simulink model "real_UIO_alternative_2021_02_17_02"  (R2019b)
settings: Solver=FixedStepAuto  StartTime=0.0  StopTime=60  FixedStep=0.01  RelTol=1e-3
values from neighbouring files (symbols this model uses):
  A = A-0.1*eye(2)    [DAC_UIO_Comp.m]    (also in LinearND_QUANTUM_2020_11_14_2.m = A+(basis{i}*rand()); UIO_adaptive_example.m = [-2379.2 0 0 0 0;0 -2.3 0 0.21 0; UIO_adaptive_example_2.m = [-1/Ta, (alpha+sigma2*wb2)/Ta, (-kb*sigma2*wb2)/Ta, -kb*sigm; UIO_adaptive_example_EEG_Balas_2ch.m = A-0.4*eye(2))
  Am = double(subs(Am_sys,{ep,Lx},{0.1,1-2*j}))    [DAC_UIO_Comp.m]    (also in UIO_adaptive_example_EEG_Balas_2ch.m = [0 1;-5 -4]; UIO_adaptive_example_alternative_EEG_ch6.m = ss_c.A; UIO_alternative_2021_01_26.m = Am-.1*eye(2); UIO_alternative_PAPER_2021_02_17.m = [0 1;-1 -1])
  B = [0;1]    [DAC_UIO_Comp.m]    (also in UIO_adaptive_example_EEG_Balas_2ch.m; UIO_adaptive_example_alternative_EEG_ch6.m = ones(opt_order,1); UIO_alternative_2021_01_26.m; UIO_alternative_PAPER_2021_02_17.m = [1;0;-1])
  C = double(subs(C_sym,{ep},{0.1}))    [DAC_UIO_Comp.m]    (also in UIO_adaptive_example.m = [1 0 0 0 0;0 0 0 1 0; 0 0 0 0 1]; UIO_adaptive_example_2.m = [1 0 0 0;0 1 0 0]; UIO_adaptive_example_EEG_Balas_2ch.m = [1, epsilon]; UIO_adaptive_example_alternative_EEG_ch6.m = ss_c.C)
  Fu = mats    [UIO_adaptive_example_alternative_EEG_ch6.m]    (also in UIO_alternative_2021_01_26.m = [0 1 ;-25 0]; UIO_alternative_PAPER_2021_02_17.m = [0,0,0,0, 0;0 0 1 0 0;0 -25 0 0 0;0 0 0 0 1;0 0 0 -144 0]; UIO_alternative_PAPER_2021_03_01.m = [0 1 0 0;-25 0 0 0;0 0 0 1;0 0 -144 0]; UIO_alternative_PAPER_2021_03_02.m = [0 1 0 0;-25 0 0 0;0 0 0 1;0 0 -144 0])
  g1 = 4+2j    [DAC_UIO_Comp.m]    (also in UIO_adaptive_example_EEG_Balas_2ch.m = 4; UIO_alternative_2021_01_26.m = 2+1j; UIO_alternative_PAPER_2021_02_17.m = 2; UIO_alternative_PAPER_2021_03_01.m = 2)
  g2 = 0    [DAC_UIO_Comp.m]    (also in UIO_adaptive_example_EEG_Balas_2ch.m = -0.3; UIO_alternative_2021_01_26.m; UIO_alternative_PAPER_2021_02_17.m = 1; UIO_alternative_PAPER_2021_03_01.m)
  g3 = 0    [DAC_UIO_Comp.m]    (also in UIO_adaptive_example_EEG_Balas_2ch.m = 0.1; UIO_alternative_2021_01_26.m; UIO_alternative_PAPER_2021_02_17.m = -3; UIO_alternative_PAPER_2021_03_01.m)
  g4 = 20    [UIO_alternative_2021_01_26.m]    (also in UIO_alternative_PAPER_2021_02_17.m = -1; UIO_alternative_PAPER_2021_03_01.m = 0; UIO_alternative_PAPER_2021_03_02.m = -2)
  gamma_e = 1    [DAC_UIO_Comp.m]    (also in UIO_adaptive_example_EEG_Balas_2ch.m; UIO_adaptive_example_alternative_EEG_ch6.m = .0001*ones(length(Am),1); UIO_alternative_2021_01_26.m = 0.001; UIO_alternative_PAPER_2021_02_17.m = 0.0001)
  K_u = ones(size(Fu,1),1)    [UIO_adaptive_example_alternative_EEG_ch6.m]    (also in UIO_alternative_2021_01_26.m = [0.215;ku]; UIO_alternative_PAPER_2021_02_17.m = [2;10;-1.6;10]; UIO_alternative_PAPER_2021_03_01.m = -[K_cvx(3:end,:)]; UIO_alternative_PAPER_2021_03_02.m)
  Theta = [real(Theta_cust);imag(Theta_cust)]    [LinearND_QUANTUM_2020_11_14_2.m]    (also in UIO_adaptive_example_alternative_EEG_ch6.m = ones(1,size(Fu,1)); UIO_alternative_2021_01_26.m = [1,1]; UIO_alternative_PAPER_2021_02_17.m = [1,1,1,1,1]; UIO_alternative_PAPER_2021_03_01.m = [1,1,1,1])
libraries: dspmtrx3 x1
settings Model: Creator=Tris  LastModifiedBy=Tris

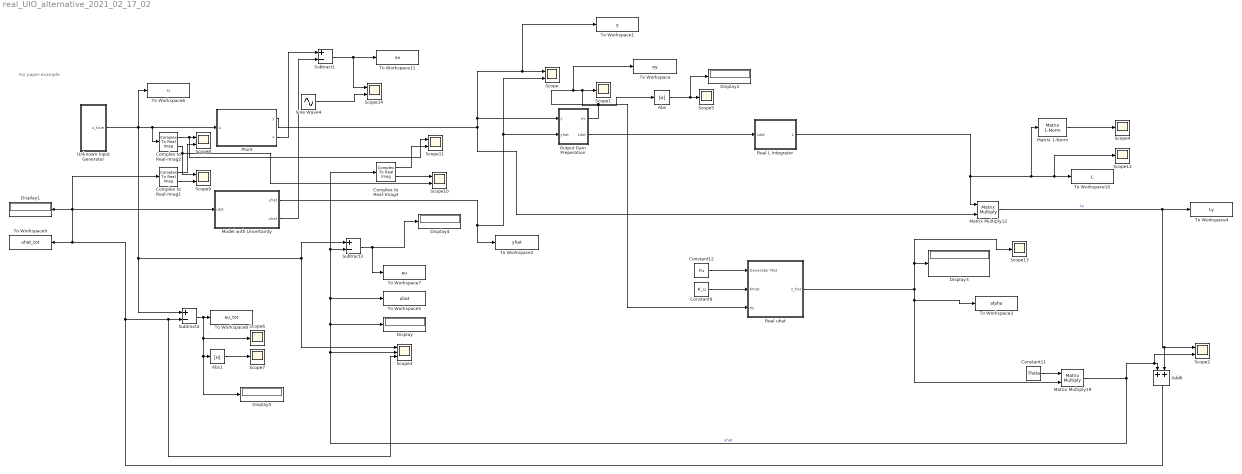
== system real_UIO_alternative_2021_02_17_02 ==
  note: For paper example
  Abs : Abs
  Abs1 : Abs
  Add6 : Sum
  Complex to Real-Imag1 : ComplexToRealImag
  Complex to Real-Imag2 : ComplexToRealImag
  Complex to Real-Imag3 : ComplexToRealImag
  Constant11 : Constant  Value=Theta  VectorParams1D=off
  Constant12 : Constant  Value=Fu
  Constant9 : Constant  Value=K_u  VectorParams1D=off
  Display{,1..5} (6 alike) : Display
  Matrix 1-Norm : dspmtrx3/Matrix  1-Norm  roundingMode=Floor  overflowMode=off  outputDataTypeStr=Inherit: Same as accumulator  outputMin=[]  outputMax=[]  outputLastDataTypeStr=Inherit: Same as accumulator
      settings: SourceProductName=DSP System Toolbox  SourceProductBaseCode=DS
  Matrix Multiply12 : Product  Multiplication=Matrix(*)
  Matrix Multiply19 : Product  Multiplication=Matrix(*)
  Model with Uncertainty : Subsystem
  Output Gain Preperation : Subsystem
  Plant : Subsystem
  Real L Integrator : Subsystem
  "Real uhat " : Subsystem
  Scope{,2,8..11,14} (7 alike) : Scope  NumInputPorts=2
  Scope{1,4..7,12..13} (7 alike) : Scope
  Scope3 : Scope  NumInputPorts=3
  Sine Wave4 : Sin  Amplitude=4  Phase=pi/2  SampleTime=0  VectorParams1D=off
  Subtract1 : Sum  Inputs=+-
  Subtract3 : Sum  Inputs=+-
  Subtract4 : Sum  Inputs=+-
  To Workspace : ToWorkspace  VariableName=ey  SaveFormat=Timeseries  SampleTime=-1
  To Workspace1 : ToWorkspace  VariableName=y  SaveFormat=Timeseries  SampleTime=-1
  To Workspace10 : ToWorkspace  VariableName=L  SaveFormat=Timeseries  SampleTime=-1
  To Workspace11 : ToWorkspace  VariableName=ex  SaveFormat=Timeseries  SampleTime=-1
  To Workspace2 : ToWorkspace  VariableName=yhat  SaveFormat=Timeseries  SampleTime=-1
  To Workspace3 : ToWorkspace  VariableName=alpha  SaveFormat=Timeseries  SampleTime=-1
  To Workspace4 : ToWorkspace  VariableName=Ly  SaveFormat=Timeseries  SampleTime=-1
  To Workspace5 : ToWorkspace  VariableName=uhat  SaveFormat=Timeseries  SampleTime=-1
  To Workspace6 : ToWorkspace  VariableName=u  SaveFormat=Timeseries  SampleTime=-1
  To Workspace7 : ToWorkspace  VariableName=eu  SaveFormat=Timeseries  SampleTime=-1
  To Workspace8 : ToWorkspace  VariableName=eu_tot  SaveFormat=Timeseries  SampleTime=-1
  To Workspace9 : ToWorkspace  VariableName=uhat_tot  SaveFormat=Timeseries  SampleTime=-1
  Unknown Input Generator : Subsystem
  wires:
  Constant11/1 -> Matrix Multiply19/1
  Matrix Multiply19/1 -> Add6/1, Scope2/2, To Workspace5/1, Complex to Real-Imag3/1, Subtract3/2, Display/1, Scope3/2  "uhat"
  Matrix Multiply12/1 -> To Workspace4/1, Add6/2, Scope2/1  "Ly"
  Constant9/1 -> "Real uhat "/2(Kmat)
  Constant12/1 -> "Real uhat "/1(Generator Mat)
  "Real uhat "/1(z_hat) -> To Workspace3/1, Matrix Multiply19/2, Scope13/1, Display3/1
  Real L Integrator/1(L) -> Matrix 1-Norm/1, Scope12/1, To Workspace10/1, Matrix Multiply12/1
  Plant/1(y) -> To Workspace1/1, Scope/1, Output Gain Preperation/1(y), Matrix Multiply12/2
  Abs/1 -> Display2/1, Scope5/1
  Unknown Input Generator/1(u_true) -> Scope3/1, Subtract3/1, Subtract4/1, To Workspace6/1, Complex to Real-Imag2/1, Plant/1(u)
  Model with Uncertainty/1(yhat) -> To Workspace2/1, Scope/2, Output Gain Preperation/2(yhat)
  Add6/1 -> Model with Uncertainty/1(utot), Complex to Real-Imag1/1, Display1/1, To Workspace9/1, Scope3/3, Subtract4/2
  Subtract3/1 -> Display4/1, To Workspace7/1
  Output Gain Preperation/1(ey) -> To Workspace/1, Abs/1, Scope1/1, "Real uhat "/3(ey)
  Output Gain Preperation/2(Ldot) -> Real L Integrator/1(Ldot)
  Abs1/1 -> Scope7/1
  Complex to Real-Imag2/1 -> Scope11/1, Scope8/1
  Complex to Real-Imag1/1 -> Scope8/2
  Complex to Real-Imag1/2 -> Scope9/2
  Complex to Real-Imag2/2 -> Scope10/2, Scope9/1
  Complex to Real-Imag3/1 -> Scope11/2
  Complex to Real-Imag3/2 -> Scope10/1
  Subtract4/1 -> Display5/1, Abs1/1, Scope6/1, To Workspace8/1
  Matrix 1-Norm/1 -> Scope4/1
  Model with Uncertainty/2(xhat) -> Subtract1/2
  Plant/2(x) -> Subtract1/1
  Subtract1/1 -> Scope14/1, To Workspace11/1
  Sine Wave4/1 -> Scope14/2

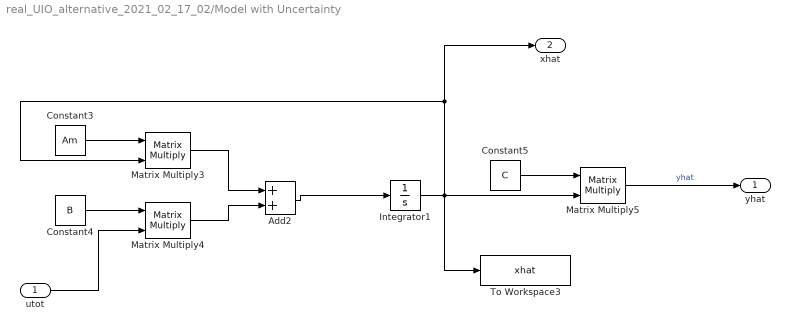
== system real_UIO_alternative_2021_02_17_02/Model with Uncertainty ==
  utot : Inport
  Add2 : Sum
  Constant3 : Constant  Value=Am
  Constant4 : Constant  Value=B  VectorParams1D=off
  Constant5 : Constant  Value=C  VectorParams1D=off
  Integrator1 : Integrator
  Matrix Multiply3 : Product  Multiplication=Matrix(*)
  Matrix Multiply4 : Product  Multiplication=Matrix(*)
  Matrix Multiply5 : Product  Multiplication=Matrix(*)
  To Workspace3 : ToWorkspace  VariableName=xhat  SaveFormat=Timeseries  SampleTime=-1
  yhat : Outport
  xhat : Outport  Port=2
  wires:
  Constant3/1 -> Matrix Multiply3/1
  Integrator1/1 -> To Workspace3/1, Matrix Multiply5/2, xhat/1, Matrix Multiply3/2
  Constant5/1 -> Matrix Multiply5/1
  Add2/1 -> Integrator1/1
  Matrix Multiply4/1 -> Add2/2
  utot/1 -> Matrix Multiply4/2
  Constant4/1 -> Matrix Multiply4/1
  Matrix Multiply3/1 -> Add2/1
  Matrix Multiply5/1 -> yhat/1  "yhat"

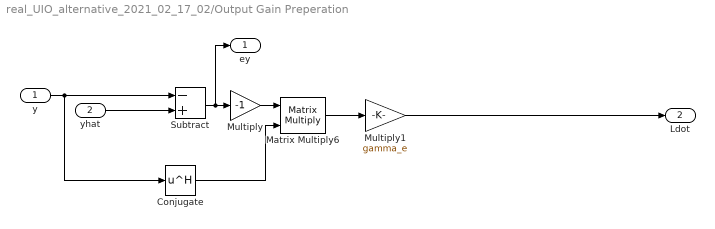
== system real_UIO_alternative_2021_02_17_02/Output Gain Preperation ==
  y : Inport
  yhat : Inport  Port=2
  Conjugate : Math  Operator=hermitian  RndMeth=Zero  SaturateOnIntegerOverflow=on
  Matrix Multiply6 : Product  Multiplication=Matrix(*)
  Multiply : Gain  Gain=-1
  Multiply1 : Gain  Gain=gamma_e
  Subtract : Sum  Inputs=-+
  ey : Outport
  Ldot : Outport  Port=2
  wires:
  Matrix Multiply6/1 -> Multiply1/1
  Multiply1/1 -> Ldot/1
  Multiply/1 -> Matrix Multiply6/1
  Conjugate/1 -> Matrix Multiply6/2
  y/1 -> Conjugate/1, Subtract/1
  yhat/1 -> Subtract/2
  Subtract/1 -> Multiply/1, ey/1

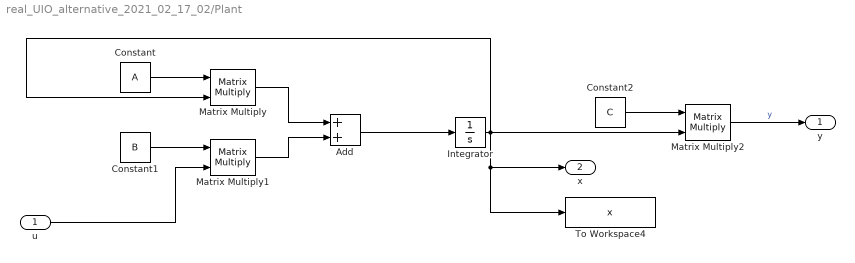
== system real_UIO_alternative_2021_02_17_02/Plant ==
  u : Inport
  Add : Sum
  Constant : Constant  Value=A
  Constant1 : Constant  Value=B  VectorParams1D=off
  Constant2 : Constant  Value=C  VectorParams1D=off
  Integrator : Integrator
  Matrix Multiply : Product  Multiplication=Matrix(*)
  Matrix Multiply1 : Product  Multiplication=Matrix(*)
  Matrix Multiply2 : Product  Multiplication=Matrix(*)
  To Workspace4 : ToWorkspace  VariableName=x  SaveFormat=Timeseries  SampleTime=-1
  y : Outport
  x : Outport  Port=2
  wires:
  Constant2/1 -> Matrix Multiply2/1
  Add/1 -> Integrator/1
  Constant1/1 -> Matrix Multiply1/1
  u/1 -> Matrix Multiply1/2
  Matrix Multiply1/1 -> Add/2
  Integrator/1 -> Matrix Multiply/2, x/1, To Workspace4/1, Matrix Multiply2/2
  Constant/1 -> Matrix Multiply/1
  Matrix Multiply/1 -> Add/1
  Matrix Multiply2/1 -> y/1  "y"

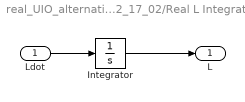
== system real_UIO_alternative_2021_02_17_02/Real L Integrator ==
  Ldot : Inport
  Integrator : Integrator  InitialCondition=0.2
  L : Outport
  wires:
  Ldot/1 -> Integrator/1
  Integrator/1 -> L/1

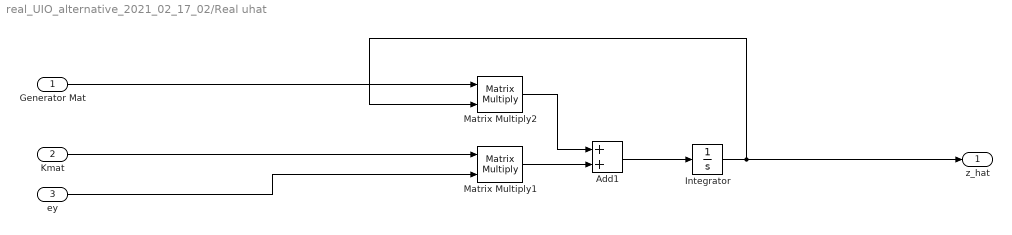
== system real_UIO_alternative_2021_02_17_02/Real uhat  ==
  Generator Mat : Inport
  Kmat : Inport  Port=2
  ey : Inport  Port=3
  Add1 : Sum
  Integrator : Integrator  InitialCondition=[-1 0 1 0]
  Matrix Multiply1 : Product  Multiplication=Matrix(*)
  Matrix Multiply2 : Product  Multiplication=Matrix(*)
  z_hat : Outport
  wires:
  ey/1 -> Matrix Multiply1/2
  Generator Mat/1 -> Matrix Multiply2/1
  Kmat/1 -> Matrix Multiply1/1
  Matrix Multiply1/1 -> Add1/2
  Add1/1 -> Integrator/1
  Matrix Multiply2/1 -> Add1/1
  Integrator/1 -> Matrix Multiply2/2, z_hat/1

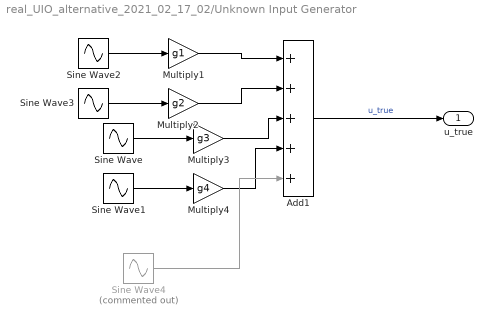
== system real_UIO_alternative_2021_02_17_02/Unknown Input Generator ==
  Add1 : Sum  Inputs=+++++
  Multiply1 : Gain  Gain=g1
  Multiply2 : Gain  Gain=g2
  Multiply3 : Gain  Gain=g3
  Multiply4 : Gain  Gain=g4
  Sine Wave : Sin  Frequency=12  SampleTime=0  VectorParams1D=off
  Sine Wave1 : Sin  Frequency=12  Phase=pi/2  SampleTime=0  VectorParams1D=off
  Sine Wave2 : Sin  Frequency=5  SampleTime=0  VectorParams1D=off
  Sine Wave3 : Sin  Frequency=5  Phase=pi/2  SampleTime=0  VectorParams1D=off
  Sine Wave4 : Sin  Commented=on  Amplitude=2  Phase=pi/2  SampleTime=0  VectorParams1D=off
  u_true : Outport
  wires:
  Multiply4/1 -> Add1/4
  Add1/1 -> u_true/1  "u_true"
  Multiply3/1 -> Add1/3
  Sine Wave/1 -> Multiply3/1
  Sine Wave1/1 -> Multiply4/1
  Multiply2/1 -> Add1/2
  Sine Wave3/1 -> Multiply2/1
  Multiply1/1 -> Add1/1
  Sine Wave2/1 -> Multiply1/1
  Sine Wave4/1 -> Add1/5
